simulink model "Sim4"  (R2021b)
settings: Solver=VariableStepAuto  StartTime=0.0  StopTime=.1  FixedStep=1e-6  RelTol=1e-6  EnableMultiTasking=on
PreLoadFcn:
  | Ts=5e-6;
InitFcn:
  | Ts=5e-6;
libraries: spsSecondOrderFilterLib x4, spsSeriesRLCBranchLib x4, spsThreePhaseVIMeasurementLib x3, spsUniversalBridgeLib x3, spsabctoAlphaBetaZeroLib x2, spsThreePhaseSeriesRLCBranchLib x2, spsAlphaBetaZerotoabcLib x1, spsPLL3phLib x1, spsabctodq0Lib x1, spsdq0toabcLib x1, spsThreePhaseSourceLib x1, spsDCVoltageSourceLib x1
settings Model: Creator=MathWorks  LastModifiedBy=sebastian
settings SolverCC: AlgebraicLoopSolver=TrustRegion  SolverResetMethod=Robust
settings DataIOCC: SaveOutput=off  SignalLogging=off  DSMLogging=off  SaveTime=off  ReturnWorkspaceOutputs=off
settings OptimizationCC: LifeSpan=inf
settings DebuggingCC: ReadBeforeWriteMsg=DisableAll  WriteAfterWriteMsg=DisableAll  WriteAfterReadMsg=DisableAll  MultiTaskDSMMsg=none  SFUnexpectedBacktrackingDiag=warning  SFNoUnconditionalDefaultTransitionDiag=warning  SFExecutionAtInitializationDiag=none  SFMachineParentedDataDiag=warning  ArithmeticOperatorsInVariantConditions=warning
settings ModelReferenceCC: UpdateModelReferenceTargets=IfOutOfDate
settings SFSimCC: SFSimEcho=off  SimUseLocalCustomCode=off  CustomCodeUndefinedFunction=UseInterfaceOnly
settings RTWCC: RTWUseLocalCustomCode=off
settings CodeAppCC: StateflowObjectComments=on
settings GRTTargetCC: TargetLangStandard=C89/C90 (ANSI)
settings ConfigComp: CovMetricSettings=dw  CovSaveCumulativeToWorkspaceVar=on  CovSaveSingleToWorkspaceVar=on  CovExternalEMLEnable=off
settings SimscapeCC: SimscapeNormalizeSystem=off  SimscapeNominalValues={1, 'bar'; 1, 'cm^3/s'; 1, 'bar*kg/s'; 1, 'kJ/kg'; 1, 'kW'; }

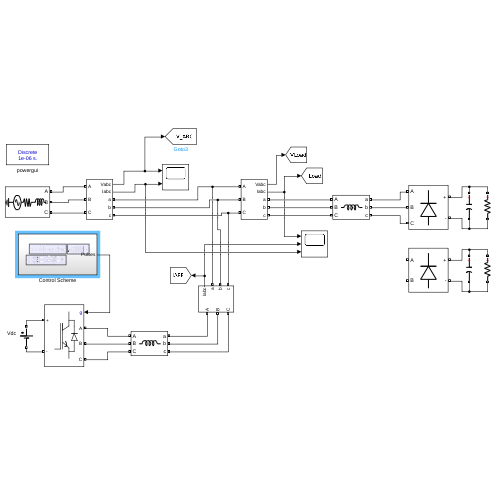
[thumbnail: Simulink's stored preview of the top-level diagram]
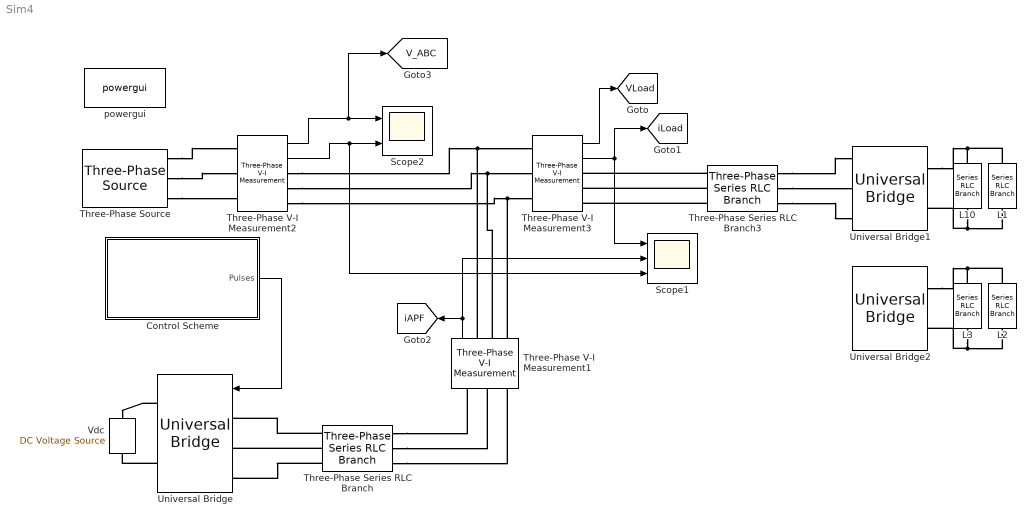
== system Sim4 ==
  Control Scheme : Subsystem
  L1 : spsSeriesRLCBranchLib/Series RLC Branch  LConnTagsString=__new0  RConnTagsString=__new0  BranchType=R  Resistance=30  Inductance=5e-4  SetiL0=off  InitialCurrent=0  Capacitance=1e-5  Setx0=off  InitialVoltage=0  Measurements=None
  L10 : spsSeriesRLCBranchLib/Series RLC Branch  LConnTagsString=__new0  RConnTagsString=__new0  BranchType=C  Resistance=1.0  Inductance=5e-4  SetiL0=off  InitialCurrent=0  Capacitance=1e-5  Setx0=off  InitialVoltage=0  Measurements=None
  L2 : spsSeriesRLCBranchLib/Series RLC Branch  LConnTagsString=__new0  RConnTagsString=__new0  BranchType=R  Resistance=30  Inductance=5e-4  SetiL0=off  InitialCurrent=0  Capacitance=1e-5  Setx0=off  InitialVoltage=0  Measurements=None
  L3 : spsSeriesRLCBranchLib/Series RLC Branch  LConnTagsString=__new0  RConnTagsString=__new0  BranchType=C  Resistance=1.0  Inductance=5e-4  SetiL0=off  InitialCurrent=0  Capacitance=1e-5  Setx0=off  InitialVoltage=0  Measurements=None
  Scope1 : Scope  NumInputPorts=3
  Scope2 : Scope  NumInputPorts=2
  Three-Phase Series RLC Branch : spsThreePhaseSeriesRLCBranchLib/Three-Phase Series RLC Branch  LConnTagsString=A|B|C  RConnTagsString=A|B|C  BranchType=L  Resistance=1  Inductance=3e-3  Capacitance=1e-6  Measurements=None
  Three-Phase Series RLC Branch3 : spsThreePhaseSeriesRLCBranchLib/Three-Phase Series RLC Branch  LConnTagsString=A|B|C  RConnTagsString=A|B|C  BranchType=L  Resistance=1  Inductance=5e-3  Capacitance=1e-6  Measurements=None
  Three-Phase V-I Measurement1 : spsThreePhaseVIMeasurementLib/Three-Phase V-I Measurement  VoltageMeasurement=no  SetLabelV=off  LabelV=Vabc  Vpu=off  VpuLL=off  CurrentMeasurement=yes  SetLabelI=off  LabelI=Iabc  Ipu=off  Pbase=100e6  Vbase=500e3  OutputType=Complex  PhasorSimulation=off  PSBequivalent=0
  Three-Phase V-I Measurement2 : spsThreePhaseVIMeasurementLib/Three-Phase V-I Measurement  VoltageMeasurement=phase-to-ground  SetLabelV=off  LabelV=Vabc  Vpu=off  VpuLL=off  CurrentMeasurement=yes  SetLabelI=off  LabelI=Iabc  Ipu=off  Pbase=100e6  Vbase=500e3  OutputType=Complex  PhasorSimulation=off  PSBequivalent=0
  Three-Phase V-I Measurement3 : spsThreePhaseVIMeasurementLib/Three-Phase V-I Measurement  VoltageMeasurement=phase-to-ground  SetLabelV=off  LabelV=Vabc  Vpu=off  VpuLL=off  CurrentMeasurement=yes  SetLabelI=off  LabelI=Iabc  Ipu=off  Pbase=100e6  Vbase=500e3  OutputType=Complex  PhasorSimulation=off  PSBequivalent=0
  Three-Phase Source : spsThreePhaseSourceLib/Three-Phase Source  InternalConnection=Yg  VoltagePhases=off  Voltage=400  PhaseAngle=0  Voltage_phases=[25e3 25e3 25e3]/sqrt(3)  PhaseAngles_phases=[0 -120 +120]  Frequency=50  NonIdealSource=on  SpecifyImpedance=on  Resistance=0.8929  Inductance=16.58e-3  ShortCircuitLevel=sqrt(3)*400*20000  BaseVoltage=400  XRratio=7  BusType=swing  Pref=10e3  Qref=0  Prefabc=[10e3, 10e3, 10e3]  Qrefabc=[0, 0, 0]  Qmin=-inf  Qmax=inf
  Universal Bridge : spsUniversalBridgeLib/Universal Bridge  Arms=3  SnubberResistance=1e5  SnubberCapacitance=inf  Device=IGBT / Diodes  Ron=1e-3  Lon=0  ForwardVoltages="[  0  0  ]"  ForwardVoltage=0  GTOparameters=[ 10e-6 , 20e-6 ]  IGBTparameters=[ 1e-6 , 2e-6 ]  Measurements=None  Measurements_2=None  converterType=Rectifier
  Universal Bridge1 : spsUniversalBridgeLib/Universal Bridge  Arms=3  SnubberResistance=500  SnubberCapacitance=250e-9  Device=Diodes  Ron=1e-3  Lon=0  ForwardVoltages="[  0  0  ]"  ForwardVoltage=0  GTOparameters=[ 10e-6 , 20e-6 ]  IGBTparameters=[ 1e-6 , 2e-6 ]  Measurements=None  Measurements_2=None  converterType=Rectifier
  Universal Bridge2 : spsUniversalBridgeLib/Universal Bridge  Arms=2  SnubberResistance=500  SnubberCapacitance=250e-9  Device=Diodes  Ron=1e-3  Lon=0  ForwardVoltages="[  0  0  ]"  ForwardVoltage=0  GTOparameters=[ 10e-6 , 20e-6 ]  IGBTparameters=[ 1e-6 , 2e-6 ]  Measurements=None  Measurements_2=None  converterType=Rectifier
  "Vdc " : spsDCVoltageSourceLib/DC Voltage Source  Amplitude=700  Measurements=None
  powergui : spspowerguiLib/powergui  Priority=1  SimulationMode=Discrete  SampleTime=1e-6  frequency=60  Iterations=50  frequencyindice=0  Pbase=100e6  ErrMax=1e-4  UnitsV=kV  UnitsW=MW  buscounter=0  FunctionMessages=off  echomessages=off  EnableUseOfTLC=off  CurrentSourceSwitches=off  DisableSnubberDevices=off  DisableRonSwitches=off  DisableVfSwitches=off  DisplayEquations=off  AutomaticDiscreteSolvers=off  SolverType=Tustin/Backward Euler (TBE)  Interpol=off  ExternalGateDelay=off  methode=off  Ts=100  x0status=blocks  SPID=off  SwTol=0  HookPort=off  NonlinearTolerance=1e-4  nMaxIteration=100  ContinueOnMaxIteration=off  RestoreLinks=warning  ResistiveCurrentMeasurement=off  Frange=[0:2:500]  Ylog=off  Xlog=on  ShowGrid=off  save=off  variable=ZData  structure=ScopeData2  ZoomFFT=off  StartTime=.07-1/50  cycles=1  DisplayStyle=1  fundamental=50  FreqAxis=off  MaxFrequency=1300  frequencyindicesteady=1  RmsSteady=1  display=off
  tag scope: VLoad=global, V_ABC=global, iAPF=global, iLoad=global
  wires:
  Three-Phase V-I Measurement2/2 -> Scope1/3, Scope2/2
  Three-Phase V-I Measurement2/1 -> [V_ABC], Scope2/1
  Three-Phase V-I Measurement3/1 -> [VLoad]
  Three-Phase V-I Measurement3/2 -> [iLoad], Scope1/1
  Control Scheme/1(Pulses) -> Universal Bridge/1
  Three-Phase V-I Measurement1/1 -> [iAPF], Scope1/2
  connections:
  Universal Bridge/RConn1 -- "Vdc "/RConn1
  Universal Bridge/RConn2 -- "Vdc "/LConn1
  Three-Phase Series RLC Branch/LConn2 -- Universal Bridge/LConn2
  Three-Phase Series RLC Branch/LConn1 -- Universal Bridge/LConn1
  Three-Phase Series RLC Branch/LConn3 -- Universal Bridge/LConn3
  Three-Phase Source/RConn3 -- Three-Phase V-I Measurement2/LConn3
  Three-Phase Source/RConn2 -- Three-Phase V-I Measurement2/LConn2
  Three-Phase Source/RConn1 -- Three-Phase V-I Measurement2/LConn1
  Three-Phase Series RLC Branch3/LConn1 -- Three-Phase V-I Measurement3/RConn1
  Three-Phase Series RLC Branch3/LConn2 -- Three-Phase V-I Measurement3/RConn2
  Three-Phase V-I Measurement2/RConn3 -- Three-Phase V-I Measurement3/LConn3 -- Three-Phase V-I Measurement1/RConn3
  Three-Phase V-I Measurement2/RConn2 -- Three-Phase V-I Measurement3/LConn2 -- Three-Phase V-I Measurement1/RConn2
  Three-Phase V-I Measurement2/RConn1 -- Three-Phase V-I Measurement1/RConn1 -- Three-Phase V-I Measurement3/LConn1
  Universal Bridge1/RConn1 -- L1/LConn1 -- L10/LConn1
  Universal Bridge1/RConn2 -- L1/RConn1 -- L10/RConn1
  Three-Phase Series RLC Branch3/RConn2 -- Universal Bridge1/LConn2
  Three-Phase Series RLC Branch/RConn1 -- Three-Phase V-I Measurement1/LConn1
  Three-Phase Series RLC Branch/RConn2 -- Three-Phase V-I Measurement1/LConn2
  Three-Phase Series RLC Branch/RConn3 -- Three-Phase V-I Measurement1/LConn3
  Three-Phase Series RLC Branch3/LConn3 -- Three-Phase V-I Measurement3/RConn3
  Three-Phase Series RLC Branch3/RConn1 -- Universal Bridge1/LConn1
  Three-Phase Series RLC Branch3/RConn3 -- Universal Bridge1/LConn3
  L3/LConn1 -- Universal Bridge2/RConn1 -- L2/LConn1
  L3/RConn1 -- Universal Bridge2/RConn2 -- L2/RConn1

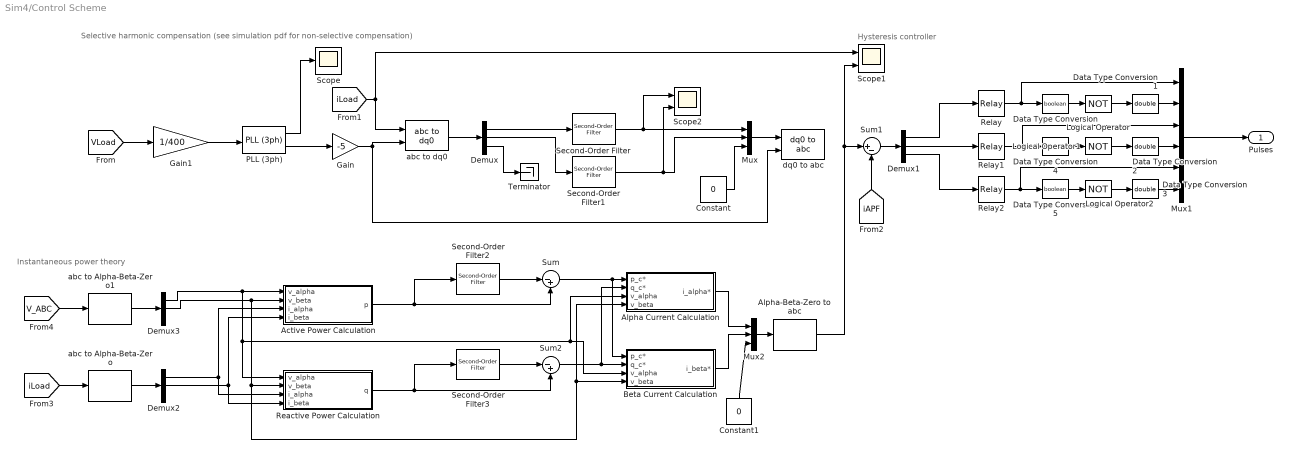
== system Sim4/Control Scheme ==
  note: Selective harmonic compensation (see simulation pdf for non-selective compensation)
  note: Hysteresis controller
  note: Instantaneous power theory
  Active Power Calculation : Subsystem
  Alpha Current Calculation : Subsystem
  Alpha-Beta-Zero to abc : spsAlphaBetaZerotoabcLib/Alpha-Beta-Zero to abc
      settings: SourceProductBaseCode=PS
  Beta Current Calculation : Subsystem
  Constant : Constant  Value=0
  Constant1 : Constant  Value=0
  Data Type Conversion : DataTypeConversion  OutDataTypeStr=boolean  SaturateOnIntegerOverflow=on  RndMeth=Zero
  Data Type Conversion1 : DataTypeConversion  OutDataTypeStr=double  SaturateOnIntegerOverflow=on  RndMeth=Zero
  Data Type Conversion2 : DataTypeConversion  OutDataTypeStr=double  SaturateOnIntegerOverflow=on  RndMeth=Zero
  Data Type Conversion3 : DataTypeConversion  OutDataTypeStr=double  SaturateOnIntegerOverflow=on  RndMeth=Zero
  Data Type Conversion4 : DataTypeConversion  OutDataTypeStr=boolean  SaturateOnIntegerOverflow=on  RndMeth=Zero
  Data Type Conversion5 : DataTypeConversion  OutDataTypeStr=boolean  SaturateOnIntegerOverflow=on  RndMeth=Zero
  Demux{,1..3} (4 alike) : Demux  Outputs=3
  Gain : Gain  Gain=-5
  Gain1 : Gain  Gain=1/400
  Logical Operator : Logic  Operator=NOT
  Logical Operator1 : Logic  Operator=NOT
  Logical Operator2 : Logic  Operator=NOT
  Mux : Mux  Inputs=3
  Mux1 : Mux  Inputs=6
  Mux2 : Mux  Inputs=3
  PLL (3ph) : spsPLL3phLib/PLL (3ph)  Fmin=45  Par_Init=[0, 50]  ParK=[180, 3200, 1]  TcD=1e-4  MaxRateChangeFreq=12  FilterCutOffFreq=25  Ts=0  AGC=on
  Reactive Power Calculation : Subsystem
  Relay : Relay  OnSwitchValue=0.1  OffSwitchValue=-0.1
  Relay1 : Relay  OnSwitchValue=0.1  OffSwitchValue=-0.1
  Relay2 : Relay  OnSwitchValue=0.1  OffSwitchValue=-0.1
  Scope : Scope
  Scope1 : Scope  NumInputPorts=2
  Scope2 : Scope  NumInputPorts=2
  Second-Order Filter : spsSecondOrderFilterLib/Second-Order Filter  FilterType=Lowpass  Fo=30  Zeta=0.707  Ts=0  Initialize=on  Vac_Init="[0,  0,  250]"  Vdc_Init=0  PlotResponse=off  FreqRange=[0, 500, 1]
      settings: SourceProductBaseCode=PS
  Second-Order Filter1 : spsSecondOrderFilterLib/Second-Order Filter  FilterType=Lowpass  Fo=30  Zeta=0.707  Ts=0  Initialize=on  Vac_Init="[0,  0,  250]"  Vdc_Init=0  PlotResponse=off  FreqRange=[0, 500, 1]
      settings: SourceProductBaseCode=PS
  Second-Order Filter2 : spsSecondOrderFilterLib/Second-Order Filter  FilterType=Lowpass  Fo=13  Zeta=0.707  Ts=0  Initialize=on  Vac_Init="[0,  0,  250]"  Vdc_Init=0  PlotResponse=off  FreqRange=[0, 500, 1]
      settings: SourceProductBaseCode=PS
  Second-Order Filter3 : spsSecondOrderFilterLib/Second-Order Filter  FilterType=Lowpass  Fo=13  Zeta=0.707  Ts=0  Initialize=on  Vac_Init="[0,  0,  250]"  Vdc_Init=0  PlotResponse=off  FreqRange=[0, 500, 1]
      settings: SourceProductBaseCode=PS
  Sum : Sum  Inputs=|-+
  Sum1 : Sum  Inputs=|+-
  Sum2 : Sum  Inputs=|-+
  Terminator : Terminator
  abc to Alpha-Beta-Zero : spsabctoAlphaBetaZeroLib/abc to Alpha-Beta-Zero
      settings: SourceProductBaseCode=PS
  abc to Alpha-Beta-Zero1 : spsabctoAlphaBetaZeroLib/abc to Alpha-Beta-Zero
      settings: SourceProductBaseCode=PS
  abc to dq0 : spsabctodq0Lib/abc to dq0  Alignment=90 degrees behind phase A axis
  dq0 to abc : spsdq0toabcLib/dq0 to abc  Alignment=90 degrees behind phase A axis
  Pulses : Outport
  wires:
  [VLoad] -> Gain1/1
  Gain1/1 -> PLL (3ph)/1
  PLL (3ph)/1 -> Scope/1
  [iLoad] -> Scope1/1, abc to dq0/1
  abc to dq0/1 -> Demux/1
  Demux/1 -> Second-Order Filter/1
  Constant/1 -> Mux/3
  Mux/1 -> dq0 to abc/1
  [iAPF] -> Sum1/2
  Mux1/1 -> Pulses/1
  Relay2/1 -> Data Type Conversion5/1, Mux1/5
  Relay1/1 -> Data Type Conversion4/1, Mux1/3
  Logical Operator2/1 -> Data Type Conversion3/1
  Data Type Conversion2/1 -> Mux1/4
  Data Type Conversion/1 -> Logical Operator/1
  Data Type Conversion3/1 -> Mux1/6
  Data Type Conversion4/1 -> Logical Operator1/1
  Logical Operator1/1 -> Data Type Conversion2/1
  Data Type Conversion5/1 -> Logical Operator2/1
  Logical Operator/1 -> Data Type Conversion1/1
  Data Type Conversion1/1 -> Mux1/2
  Relay/1 -> Data Type Conversion/1, Mux1/1
  Demux1/2 -> Relay1/1
  Demux1/1 -> Relay/1
  Demux1/3 -> Relay2/1
  Sum1/1 -> Demux1/1
  Demux/3 -> Terminator/1
  Gain/1 -> abc to dq0/2, dq0 to abc/2
  Demux/2 -> Second-Order Filter1/1
  Second-Order Filter1/1 -> Scope2/2, Mux/2
  Second-Order Filter/1 -> Scope2/1, Mux/1
  [iLoad] -> abc to Alpha-Beta-Zero/1
  PLL (3ph)/2 -> Gain/1
  [V_ABC] -> abc to Alpha-Beta-Zero1/1
  abc to Alpha-Beta-Zero/1 -> Demux2/1
  abc to Alpha-Beta-Zero1/1 -> Demux3/1
  Demux3/1 -> Beta Current Calculation/3(v_alpha), Alpha Current Calculation/3(v_alpha), Reactive Power Calculation/1(v_alpha), Active Power Calculation/1(v_alpha)
  Demux3/2 -> Alpha Current Calculation/4(v_beta), Beta Current Calculation/4(v_beta), Reactive Power Calculation/2(v_beta), Active Power Calculation/2(v_beta)
  Demux2/1 -> Reactive Power Calculation/3(i_alpha), Active Power Calculation/3(i_alpha)
  Active Power Calculation/1(p) -> Sum/2, Second-Order Filter2/1
  Second-Order Filter2/1 -> Sum/1
  Second-Order Filter3/1 -> Sum2/1
  Reactive Power Calculation/1(q) -> Second-Order Filter3/1, Sum2/2
  Sum/1 -> Alpha Current Calculation/1(p_c*), Beta Current Calculation/1(p_c*)
  Sum2/1 -> Alpha Current Calculation/2(q_c*), Beta Current Calculation/2(q_c*)
  Mux2/1 -> Alpha-Beta-Zero to abc/1
  Alpha Current Calculation/1(i_alpha*) -> Mux2/1
  Beta Current Calculation/1(i_beta*) -> Mux2/2
  Constant1/1 -> Mux2/3
  Demux2/2 -> Reactive Power Calculation/4(i_beta), Active Power Calculation/4(i_beta)
  Alpha-Beta-Zero to abc/1 -> Sum1/1, Scope1/2

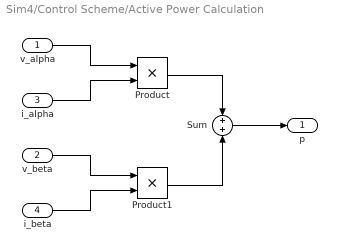
== system Sim4/Control Scheme/Active Power Calculation ==
  v_alpha : Inport
  v_beta : Inport  Port=2
  i_alpha : Inport  Port=3
  i_beta : Inport  Port=4
  Product : Product
  Product1 : Product
  Sum : Sum  Inputs=+|+
  p : Outport
  wires:
  v_alpha/1 -> Product/1
  i_alpha/1 -> Product/2
  v_beta/1 -> Product1/1
  i_beta/1 -> Product1/2
  Product/1 -> Sum/1
  Product1/1 -> Sum/2
  Sum/1 -> p/1

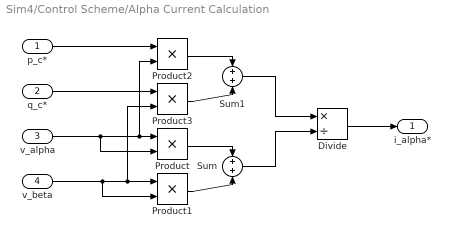
== system Sim4/Control Scheme/Alpha Current Calculation ==
  p_c* : Inport
  q_c* : Inport  Port=2
  v_alpha : Inport  Port=3
  v_beta : Inport  Port=4
  Divide : Product  Inputs=*/
  Product{,1..3} (4 alike) : Product
  Sum : Sum  Inputs=+|+
  Sum1 : Sum  Inputs=+|+
  i_alpha* : Outport
  wires:
  v_alpha/1 -> Product/2, Product2/2, Product/1
  v_beta/1 -> Product1/2, Product3/2, Product1/1
  Product/1 -> Sum/1
  Product1/1 -> Sum/2
  Sum/1 -> Divide/2
  Divide/1 -> i_alpha*/1
  p_c*/1 -> Product2/1
  q_c*/1 -> Product3/1
  Product3/1 -> Sum1/2
  Product2/1 -> Sum1/1
  Sum1/1 -> Divide/1

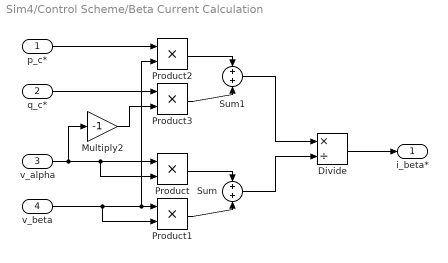
== system Sim4/Control Scheme/Beta Current Calculation ==
  p_c* : Inport
  q_c* : Inport  Port=2
  v_alpha : Inport  Port=3
  v_beta : Inport  Port=4
  Divide : Product  Inputs=*/
  Multiply2 : Gain  Gain=-1
  Product{,1..3} (4 alike) : Product
  Sum : Sum  Inputs=+|+
  Sum1 : Sum  Inputs=+|+
  i_beta* : Outport
  wires:
  v_alpha/1 -> Product/2, Product/1, Multiply2/1
  v_beta/1 -> Product1/2, Product2/2, Product1/1
  Product/1 -> Sum/1
  Product1/1 -> Sum/2
  Sum/1 -> Divide/2
  Divide/1 -> i_beta*/1
  p_c*/1 -> Product2/1
  q_c*/1 -> Product3/1
  Product3/1 -> Sum1/2
  Product2/1 -> Sum1/1
  Sum1/1 -> Divide/1
  Multiply2/1 -> Product3/2

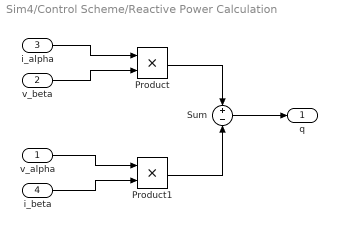
== system Sim4/Control Scheme/Reactive Power Calculation ==
  v_alpha : Inport
  v_beta : Inport  Port=2
  i_alpha : Inport  Port=3
  i_beta : Inport  Port=4
  Product : Product
  Product1 : Product
  Sum : Sum  Inputs=+|-
  q : Outport
  wires:
  Product/1 -> Sum/1
  Product1/1 -> Sum/2
  Sum/1 -> q/1
  i_alpha/1 -> Product/1
  v_beta/1 -> Product/2
  v_alpha/1 -> Product1/1
  i_beta/1 -> Product1/2
